simulink model "SimulinkPacer"  (R2022a)
settings: Solver=FixedStepAuto  StartTime=0.0  StopTime=10.0  FixedStep=1e-3  RelTol=1e-3  EnableMultiTasking=on
undefined symbols (not defined in the file): D10, D11, D12, D13, D2, D4, D5, D7, D8, D9, PTA0, PTA2, PTB23, PTB9, PTC3, PTC4, PTD0, PTD1, PTD2, PTD3
libraries: frdmk64flib x12
settings Model: ExtModeTrigDuration=5  Creator=sabri  LastModifiedBy=sabri
settings SolverCC: AlgebraicLoopSolver=TrustRegion
settings OptimizationCC: EnhancedBackFolding=on  PassReuseOutputArgsAs=Individual arguments  ZeroExternalMemoryAtStartup=off  ZeroInternalMemoryAtStartup=off  MaxStackSize=64  OptimizeBlockOrder=speed  DifferentSizesBufferReuse=on  OptimizationCustomize=off  EfficientTunableParamExpr=on
settings DebuggingCC: ParameterTunabilityLossMsg=error  UnconnectedInputMsg=warning  UnconnectedOutputMsg=warning  UnconnectedLineMsg=warning  SFMachineParentedDataDiag=warning
settings HardwareCC: ProdBitPerPointer=32  ProdBitPerSizeT=32  ProdBitPerPtrDiffT=32  ProdLargestAtomicInteger=Long  ProdLargestAtomicFloat=Double  ProdWordSize=32  ProdHWDeviceType=ARM Compatible->ARM Cortex
settings SFSimCC: MATLABDynamicMemAlloc=off
settings RTWCC: SystemTargetFile=ert.tlc  HardwareBoard=NXP FRDM-K64F  TLCOptions="-aInlineSetEventsForThisBaseRateFcn=TLC_FALSE -aSuppressMultiTaskScheduler=TLC_FALSE  -aRateBasedStepFcn=0"  TemplateMakefile=ert_default_tmf  Toolchain=GNU Tools for ARM Embedded Processors
settings CodeAppCC: ForceParamTrailComments=on  IgnoreCustomStorageClasses=off  OperatorAnnotations=on  SimulinkDataObjDesc=on  SFDataObjDesc=on  InsertBlockDesc=on

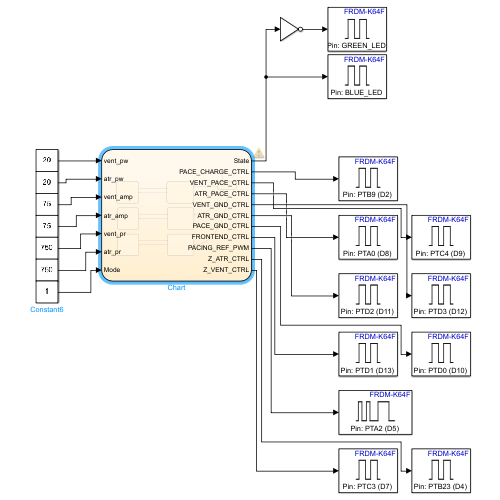
[thumbnail: Simulink's stored preview of the top-level diagram]
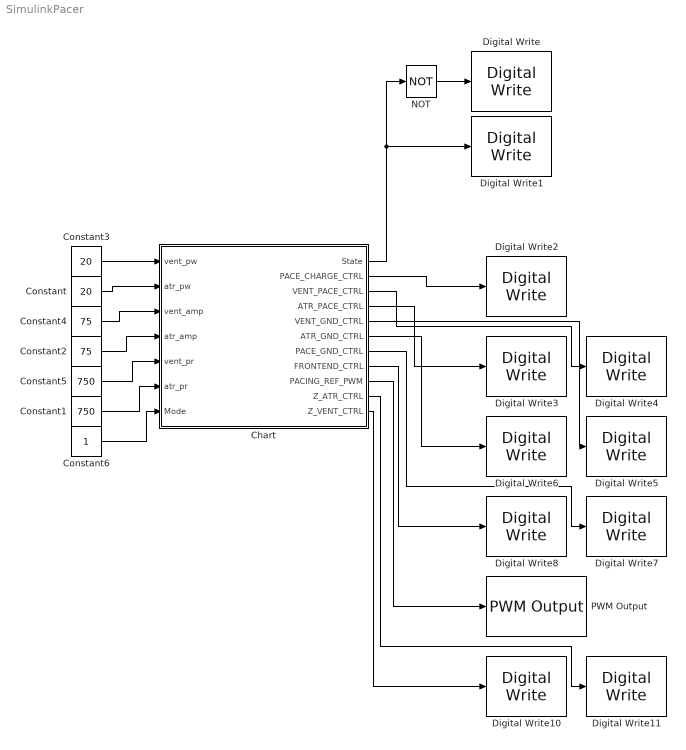
== system SimulinkPacer ==
  Chart : Stateflow chart  TreatAsAtomicUnit=on
  Constant : Constant  Value=20
  Constant1 : Constant  Value=750
  Constant2 : Constant  Value=75
  Constant3 : Constant  Value=20
  Constant4 : Constant  Value=75
  Constant5 : Constant  Value=750
  Constant6 : Constant
  Digital Write : frdmk64flib/Digital Write  Whichpin=GREEN_LED
  Digital Write1 : frdmk64flib/Digital Write  Whichpin=BLUE_LED
  Digital Write10 : frdmk64flib/Digital Write  Whichpin=PTC3 (D7)
  Digital Write11 : frdmk64flib/Digital Write  Whichpin=PTB23 (D4)
  Digital Write2 : frdmk64flib/Digital Write  Whichpin=PTB9 (D2)
  Digital Write3 : frdmk64flib/Digital Write  Whichpin=PTA0 (D8)
  Digital Write4 : frdmk64flib/Digital Write  Whichpin=PTC4 (D9)
  Digital Write5 : frdmk64flib/Digital Write  Whichpin=PTD3 (D12)
  Digital Write6 : frdmk64flib/Digital Write  Whichpin=PTD2 (D11)
  Digital Write7 : frdmk64flib/Digital Write  Whichpin=PTD0 (D10)
  Digital Write8 : frdmk64flib/Digital Write  Whichpin=PTD1 (D13)
  NOT : Logic  Operator=NOT  IconShape=distinctive  AllPortsSameDT=off  OutDataTypeStr=boolean
  PWM Output : frdmk64flib/PWM Output  Whichpin=PTA2 (D5)  InitialFrequency=2000  InitialDutyCycle=0
  wires:
  Constant/1 -> Chart/2(atr_pw)
  Constant1/1 -> Chart/6(atr_pr)
  Constant2/1 -> Chart/4(atr_amp)
  Constant3/1 -> Chart/1(vent_pw)
  Constant4/1 -> Chart/3(vent_amp)
  NOT/1 -> Digital Write/1
  Chart/2(PACE_CHARGE_CTRL) -> Digital Write2/1
  Chart/3(VENT_PACE_CTRL) -> Digital Write4/1
  Chart/4(ATR_PACE_CTRL) -> Digital Write3/1
  Chart/6(ATR_GND_CTRL) -> Digital Write6/1
  Chart/8(FRONTEND_CTRL) -> Digital Write8/1
  Chart/7(PACE_GND_CTRL) -> Digital Write7/1
  Chart/9(PACING_REF_PWM) -> PWM Output/1
  Constant5/1 -> Chart/5(vent_pr)
  Chart/1(State) -> Digital Write1/1, NOT/1
  Chart/5(VENT_GND_CTRL) -> Digital Write5/1
  Chart/10(Z_ATR_CTRL) -> Digital Write11/1
  Chart/11(Z_VENT_CTRL) -> Digital Write10/1
  Constant6/1 -> Chart/7(Mode)

== stateflow chart SimulinkPacer/Chart ==
  state VOO_Pacing
    entry:
    State = 1
    PACE_CHARGE_CTRL = 0
    PACE_GND_CTRL = 1
    ATR_PACE_CTRL = 0
    ATR_GND_CTRL = 0
    Z_ATR_CTRL = 0
    Z_VENT_CTRL = 0
    VENT_GND_CTRL = 0
    VENT_PACE_CTRL = 1
    FRONTEND_CTRL = 0
    PACING_REF_PWM = vent_amp
  state VOO_Charging
    entry:
    State = 0
    PACE_GND_CTRL = 1
    VENT_PACE_CTRL = 0
    Z_ATR_CTRL = 0
    Z_VENT_CTRL = 0
    ATR_GND_CTRL = 0
    VENT_GND_CTRL = 1
    ATR_PACE_CTRL = 0
    PACING_REF_PWM = vent_amp
    PACE_CHARGE_CTRL = 1
    FRONTEND_CTRL = 0
  state ModeSelect
  state AOO_Pacing
    entry:
    State = 1
    PACE_CHARGE_CTRL = 0
    PACE_GND_CTRL = 1
    ATR_PACE_CTRL = 1
    ATR_GND_CTRL = 0
    Z_ATR_CTRL = 0
    Z_VENT_CTRL = 0
    VENT_GND_CTRL = 0
    VENT_PACE_CTRL = 0
    FRONTEND_CTRL = 0
    PACING_REF_PWM = atr_amp
  state AOO_Charging
    entry:
    State = 0
    PACE_GND_CTRL = 1
    VENT_PACE_CTRL = 0
    Z_ATR_CTRL = 0
    Z_VENT_CTRL = 0
    ATR_GND_CTRL = 1
    VENT_GND_CTRL = 0
    ATR_PACE_CTRL = 0
    PACING_REF_PWM = atr_amp
    PACE_CHARGE_CTRL = 1
    FRONTEND_CTRL = 0
  state VII_Pacing
    entry:
    State = 1
    PACE_CHARGE_CTRL = 0
    PACE_GND_CTRL = 1
    ATR_PACE_CTRL = 0
    ATR_GND_CTRL = 0
    Z_ATR_CTRL = 0
    Z_VENT_CTRL = 0
    VENT_GND_CTRL = 0
    VENT_PACE_CTRL = 1
    FRONTEND_CTRL = 0
    PACING_REF_PWM = vent_amp
  state VII_Charging
    entry:
    State = 0
    PACE_GND_CTRL = 1
    VENT_PACE_CTRL = 0
    Z_ATR_CTRL = 0
    Z_VENT_CTRL = 0
    ATR_GND_CTRL = 0
    VENT_GND_CTRL = 1
    ATR_PACE_CTRL = 0
    PACING_REF_PWM = vent_amp
    PACE_CHARGE_CTRL = 1
    FRONTEND_CTRL = 0
  (default) -> ModeSelect
  ModeSelect -> VOO_Charging [order 1] : [Mode == 1]
  VOO_Pacing -> VOO_Charging : [after(vent_pw, msec)]
  ModeSelect -> VII_Charging [order 3] : [Mode == 3]
  ModeSelect -> AOO_Charging [order 2] : [Mode == 2]
  VOO_Charging -> VOO_Pacing : [after(vent_pr - vent_pw, msec)]
  AOO_Pacing -> AOO_Charging : [after(atr_pw, msec)]
  AOO_Charging -> AOO_Pacing : [after(atr_pr - atr_pw, msec)]
  VII_Pacing -> VII_Charging : [after(vent_pw, msec)]
  VII_Charging -> VII_Pacing : [after(vent_pr - vent_pw, msec)]
  data: vent_pw input; atr_pw input; vent_amp input; atr_amp input; vent_pr input; atr_pr input; State output double =0; PACE_CHARGE_CTRL output; VENT_PACE_CTRL output; ATR_PACE_CTRL output; VENT_GND_CTRL output; ATR_GND_CTRL output; PACE_GND_CTRL output; FRONTEND_CTRL output; PACING_REF_PWM output; Z_ATR_CTRL output; Z_VENT_CTRL output; Mode input
